simulink model "exemplo_simulink"  (R2015a)
settings: Solver=ode45  StartTime=0.0  StopTime=10.0  RelTol=1e-3
libraries: simulink x1
settings Model: Creator=buging  LastModifiedBy=buging

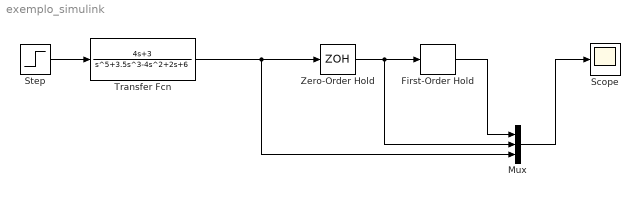
== system exemplo_simulink ==
  First-Order Hold : simulink/Discrete/First-Order Hold  DisableCoverage=on  Ts=0.3
  Mux : Mux  Inputs=3
  Scope : Scope
  Step : Step  SampleTime=0
  Transfer Fcn : TransferFcn  Numerator=[4 3]  Denominator=[1 0 3.5 -4 2 6]
  Zero-Order Hold : ZeroOrderHold  SampleTime=0.3
  wires:
  Step/1 -> Transfer Fcn/1
  Zero-Order Hold/1 -> Mux/2, First-Order Hold/1
  Transfer Fcn/1 -> Mux/3, Zero-Order Hold/1
  Mux/1 -> Scope/1
  First-Order Hold/1 -> Mux/1
